simulink model "NHTSA_LDW_Curved_dashed_right_cs"  (Simulink 7.6)
settings: Solver=ode5  SolverMode=SingleTasking  StartTime=0.0  StopTime=10  FixedStep=1/100  RelTol=1e-3
model workspace (MAT data in the model file):
  mbox_table : struct (value not decoded)
  model_closed = 0
  sim_status = 0
PreLoadFcn:
  | check_NUTS_defined;
  | 
  | assignin('base',['model_closed_' bdroot],false);
  | 
  | if exist('LDW_mask_sfun.mexw64')==3
  | delete LDW_mask_sfun.mexw64;
  | end
  | 
  | if exist('LDW_mask_sfun.mexw32') ==3
  | delete LDW_mask_sfun.mexw32;
  | end
  | 
  | switch version('-release')
  | case {'2010a', '2010b', '2011a'}
  | addpath('../includes_LKAS/includes_LKAS_2010a');
  | case {'2011b', '2012a', '2012b'}
  | addpath('../includes_LKAS/includes_LKAS_2011b');
  | otherwise
  | addpath('../includes_LKAS/includes_LKAS_2011b');
  | end
InitFcn:
  | PreScanExperimentInitFcn(bdroot)
StopFcn:
  | PreScanExperimentStopFcn(bdroot)
undefined symbols (not defined in the file): DiscIntNeverNeededParam, InitImageOutputDir, x_ini_VRML, y_ini_VRML, z_ini_VRML
libraries: simulink x22, PreScanSimulinkLibrary x7, simulink_extras x6, dspsnks4 x2, PreScanUsefulBlocks x2, simulink_need_slupdate x1
(part 1 of 5)
CloseFcn:
  | evalin('base',['clear model_closed_' bdroot]);
  | 
  | set(0, 'ShowHiddenHandles', 'on')
  | 
  | try
  |     close (PlotSpeed)
  | end
  | 
  | try
  |     close(findobj('Name','Filtered'))
  | end
  | 
  | try
  |     close(findobj('Name','Results'))
  | end
  | 
  | set(0, 'ShowHiddenHandles', 'off')
settings Model: Creator=PRESCAN  LastModifiedBy=buildbot
settings OptimizationCC: InitFltsAndDblsToZero=on
settings DebuggingCC: SaveWithParameterizedLinksMsg=none  SignalResolutionControl=TryResolveAllWithWarning  SolverPrmCheckMsg=none  MultiTaskDSMMsg=warning  MultiTaskCondExecSysMsg=none
settings SFSimCC: SimParseCustomCode=off
settings RTWCC: IncludeERTFirstTime=on
settings GRTTargetCC: TargetFcnLib=ansi_tfl_tmw.mat

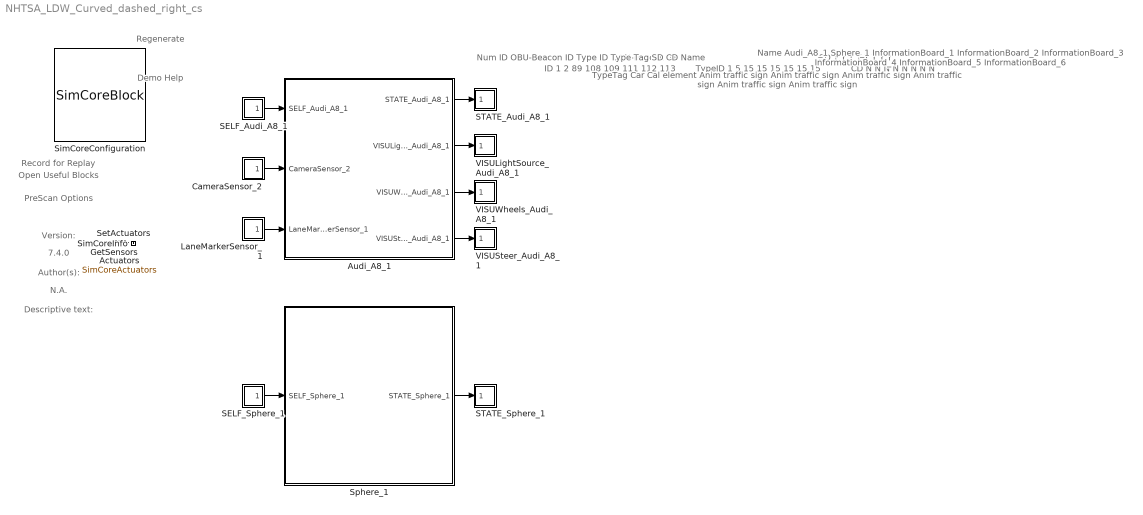
== system NHTSA_LDW_Curved_dashed_right_cs ==
  note: Demo Help
  note: Regenerate
  note: Record for Replay
  note: Open Useful Blocks
  note: PreScan Options
  note: Version:
  note: 7.4.0
  note: Author(s):
  note: N.A.
  note: Descriptive text:
  note: ID
      |
      | 1
      | 2
      | 89
      | 108
      | 109
      | 111
      | 112
      | 113
  note: OBU-Beacon ID
  note: TypeID
      |
      | 1
      | 5
      | 15
      | 15
      | 15
      | 15
      | 15
      | 15
  note: TypeTag
      |
      | Car
      | Cal element
      | Anim traffic sign
      | Anim traffic sign
      | Anim traffic sign
      | Anim traffic sign
      | Anim traffic sign
      | Anim traffic sign
  note: SD
      |
      | Y
      | Y
      | Y
      | Y
      | Y
      | Y
      | Y
      | Y
  note: CD
      |
      | N
      | N
      | N
      | N
      | N
      | N
      | N
      | N
  note: Name
      |
      | Audi_A8_1
      | Sphere_1
      | InformationBoard_1
      | InformationBoard_2
      | InformationBoard_3
      | InformationBoard_4
      | InformationBoard_5
      | InformationBoard_6
  note: Num ID OBU-Beacon ID Type ID Type Tag SD CD Name
  Actuators : DataStoreMemory  Tag=Actuators  DataStoreName=SimCoreActuators  InitialValue=zeros(258,1)
      settings: DeleteFcn=PreScanBlockDeleteFcn;
  Audi_A8_1 : Subsystem  Tag=WorldObjectSubSystem  InitFcn=UniqueId = '253';
      mask Display: image(imread('Audi_A8.jpg'));color('white');text(0,0,' ID=1\n')
  CameraSensor_2 : Subsystem  Tag=CameraSensor  Priority=3
      settings: DeleteFcn=PreScanBlockDeleteFcn;
      mask Type: PreScan Source Block: Camera Sensor
      mask Description: The Camera Sensor provides a color or monochrome image.
      mask Help: eval('openHelp(457)')
      mask Display: image(imread('CameraSensor.png'))
  GetSensors : Subsystem  Tag=GetSensors  Priority=2  mask(PreScan Simulation Core Block){NrOfSensors=16, TimeStep=1/100}
      mask prompts: NrOfSensors "Number of sensor values"; TimeStep "Timestep [s]"
      mask help:
      | Please do not remove this block from the PreScan compilation sheet,
      | as it contains essential configuration parameters for a PreScan simulation.
      settings: DeleteFcn=PreScanBlockDeleteFcn;
  LaneMarkerSensor_1 : Subsystem  Tag=LaneMarkerSensor  Priority=3
      settings: DeleteFcn=PreScanBlockDeleteFcn;
      mask Type: PreScan Source Block: Lane Marker Sensor
      mask Description: The Lane Marker Sensor provides information relating the sensor to the lane markers on the road.
      mask Help: eval('openHelp(457)')
      mask Display: image(imread('LaneMarkerSensorSL.png'))
  SELF_Audi_A8_1 : Subsystem  Tag=SELF  Priority=3  mask(PreScan Source Block: SELF){PortName=SELF_Audi_A8_1, PortIndex=0, PortWidth=8, TimeStep=1/100}
      mask prompts: PortName "Auto-Assigned: Port Name [-]"; PortIndex "Auto-Assigned: Port Index [-]"; PortWidth "Auto-Assigned: Port Dimensions"; TimeStep "Auto-Assigned: Upload Period [s]"
      mask help:
      | The SELF port shows (state) information of the actor itself. The outputs are position in the experiment's axis system and the GPS coordinates, and the object's absolute velocity and compass heading.
      |
      | For more information, please click Help.
      settings: DeleteFcn=PreScanBlockDeleteFcn;
      mask Help: eval('openHelp(462)')
      mask Display: image(imread('GPS.png'))
  SELF_Sphere_1 : Subsystem  Tag=SELF  Priority=3  mask(PreScan Source Block: SELF){PortName=SELF_Sphere_1, PortIndex=8, PortWidth=8, TimeStep=1/100}
      mask prompts: PortName "Auto-Assigned: Port Name [-]"; PortIndex "Auto-Assigned: Port Index [-]"; PortWidth "Auto-Assigned: Port Dimensions"; TimeStep "Auto-Assigned: Upload Period [s]"
      mask help:
      | The SELF port shows (state) information of the actor itself. The outputs are position in the experiment's axis system and the GPS coordinates, and the object's absolute velocity and compass heading.
      |
      | For more information, please click Help.
      settings: DeleteFcn=PreScanBlockDeleteFcn;
      mask Help: eval('openHelp(462)')
      mask Display: image(imread('GPS.png'))
  STATE_Audi_A8_1 : Subsystem  Tag=State  Priority=0  mask(PreScan Sink Block: State){x0=25.564167022705078, y0=61.75, z0=0.55, Roll0=0, Pitch0=0, Yaw0=0, TimeStep=1/100}
      mask prompts: x0 "Ini x-position VEHICLE wrt GLOBAL axis system [m]"; y0 "Ini y-position VEHICLE wrt GLOBAL axis system [m]"; z0 "Ini z-position VEHICLE wrt GLOBAL axis system [m]"; Roll0 "Ini roll-angle BODY wrt VEHICLE axis system [deg]"; Pitch0 "Ini pitch-angle BODY wrt VEHICLE axis system [deg]"; Yaw0 "Ini yaw-angle VEHICLE wrt GLOBAL axis system [deg]"; TimeStep "Time Step [s]"
      mask help:
      | The Actor State contains a vector signal of size (9x1), containing the following signals:
      |
      | -  Position                  (x,y,z)                                     [m]
      | -  Velocity                  (vx,vy,vz)                               [m/s]
      | -  Angles                    (Roll, Pitch, Yaw)                   [rad]
      |
      | The Actor state is defined in the global axis system.
      | The state is superponed on the Initial position defined in the GUI.
      |
      | For more information, please click Help.
      settings: DeleteFcn=PreScanBlockDeleteFcn;
      mask Help: eval('openHelp(222)')
      mask Display: image(imread('State.png'))
  STATE_Sphere_1 : Subsystem  Tag=State  Priority=0  mask(PreScan Sink Block: State){x0=25.564167022705078, y0=61.75, z0=0, Roll0=0, Pitch0=0, Yaw0=0, TimeStep=1/100}
      mask prompts: x0 "Ini x-position VEHICLE wrt GLOBAL axis system [m]"; y0 "Ini y-position VEHICLE wrt GLOBAL axis system [m]"; z0 "Ini z-position VEHICLE wrt GLOBAL axis system [m]"; Roll0 "Ini roll-angle BODY wrt VEHICLE axis system [deg]"; Pitch0 "Ini pitch-angle BODY wrt VEHICLE axis system [deg]"; Yaw0 "Ini yaw-angle VEHICLE wrt GLOBAL axis system [deg]"; TimeStep "Time Step [s]"
      mask help:
      | The Actor State contains a vector signal of size (9x1), containing the following signals:
      |
      | -  Position                  (x,y,z)                                     [m]
      | -  Velocity                  (vx,vy,vz)                               [m/s]
      | -  Angles                    (Roll, Pitch, Yaw)                   [rad]
      |
      | The Actor state is defined in the global axis system.
      | The state is superponed on the Initial position defined in the GUI.
      |
      | For more information, please click Help.
      settings: DeleteFcn=PreScanBlockDeleteFcn;
      mask Help: eval('openHelp(222)')
      mask Display: image(imread('State.png'))
  SetActuators : Subsystem  Tag=SetActuators  Priority=1  mask(PreScan Simulation Core Block){TimeStep=1/100, NrOfActuators=258}
      mask prompts: TimeStep "Timestep [s]"; NrOfActuators "Number of actuator values"
      mask help:
      | Please do not remove this block from the PreScan compilation sheet,
      | as it contains essential configuration parameters for a PreScan simulation.
      settings: DeleteFcn=PreScanBlockDeleteFcn;
  SimCoreConfiguration : M-S-Function  Tag=SimCoreConfiguration  Description=7FB4F5B2D4E922D3E47F677EE9558725FCFBD13CCF8702ED0EADB85902E5BDE3  FunctionName=SimCoreBlock  Parameters=ExperimentXML PortsXML SimulationCore HostName CheckStart EnableLog RfR EnableGPUAccel ShowComputationTime  mask(PreScan Simulation Core Configurator){SimulationCore=NUTS, HostName=0, CheckStart=0, prescanversion='7.4.0', EnableLog=off, RfR=0, EnableGPUAccel=off, ShowComputationTime=off}
      mask prompts: SimulationCore "Simulation Core"; HostName "Simulation Host"; CheckStart "Show START Dialog"; prescanversion "PreScan Version"; EnableLog "Create TA Log"; RfR "Record for Replay"; EnableGPUAccel "Enable GPU Acceleration"; ShowComputationTime "Show ComputationTime Scope"
      mask help:
      | Please do not remove this block from the PreScan compilation sheet,
      | as it contains essential configuration parameter for a PreScan simulation.
      mask init:
      | model = bdroot;
      | ExperimentXML = [model(1:end-3) '.pex'];
      | PortsXML = [model '_ports.pcd'];
      settings: DeleteFcn=PreScanBlockDeleteFcn;  ModelCloseFcn=assignin('base',['model_closed_' bdroot],true);
      mask Help: eval('openHelp(812)')
      mask Display: image(imread('prescanlogo.ico'))
  SimCoreInfo : Subsystem  Tag=SimCoreInfo
  Sphere_1 : Subsystem  Tag=WorldObjectSubSystem  InitFcn=UniqueId = '274';
      mask Display: image(imread('Sphere.jpg'));color('white');text(0,0,' ID=2\n')
  VISULightSource_Audi_A8_1 : Subsystem  Tag=VisuLightSource  Priority=0
      settings: DeleteFcn=PreScanBlockDeleteFcn;
      mask Type: PreScan Sink Block: VisuLightSource
      mask Description:
      | The VisuLightSource block provides a way to animate Light Sources of the indicator, braking, fog and main lights of a vehicle.
      | 
      | For more information, please click Help.
      mask Help: eval('openHelp(223)')
      mask Display: image(imread('RearLight.png'))
  VISUSteer_Audi_A8_1 : Subsystem  Tag=VisuSteer  Priority=0
      settings: DeleteFcn=PreScanBlockDeleteFcn;
      mask Type: PreScan Sink Block: VisuSteer
      mask Description:
      | The VisuSteer block provides a way to adapt the orientation of the steering column and steering wheel of a vehicle.
      | 
      | For more information, please click Help.
      mask Help: eval('openHelp(223)')
      mask Display: image(imread('steeringwheel.png'))
  VISUWheels_Audi_A8_1 : Subsystem  Tag=VisuWheels  Priority=0
      settings: DeleteFcn=PreScanBlockDeleteFcn;
      mask Type: PreScan Sink Block: VisuWheels
      mask Description:
      | The VisuWheels block provides a way to animate the wheels of a vehicle, with steering, rotation (because of velocity) and z-displacement.
      | 
      | For more information, please click Help.
      mask Help: eval('openHelp(223)')
      mask Display: image(imread('wheel.png'))
  wires:
  Audi_A8_1/1(STATE_Audi_A8_1) -> STATE_Audi_A8_1/1(State)
  SELF_Audi_A8_1/1(U) -> Audi_A8_1/1(SELF_Audi_A8_1)
  CameraSensor_2/1(U1) -> Audi_A8_1/2(CameraSensor_2)
  LaneMarkerSensor_1/1(U) -> Audi_A8_1/3(LaneMarkerSensor_1)
  Audi_A8_1/2(VISULightSource_Audi_A8_1) -> VISULightSource_Audi_A8_1/1(Lights)
  Audi_A8_1/3(VISUWheels_Audi_A8_1) -> VISUWheels_Audi_A8_1/1(Wheels)
  Audi_A8_1/4(VISUSteer_Audi_A8_1) -> VISUSteer_Audi_A8_1/1(Steer)
  Sphere_1/1(STATE_Sphere_1) -> STATE_Sphere_1/1(State)
  SELF_Sphere_1/1(U) -> Sphere_1/1(SELF_Sphere_1)
  SetActuators/1(dummy) -> GetSensors/1(dummy)

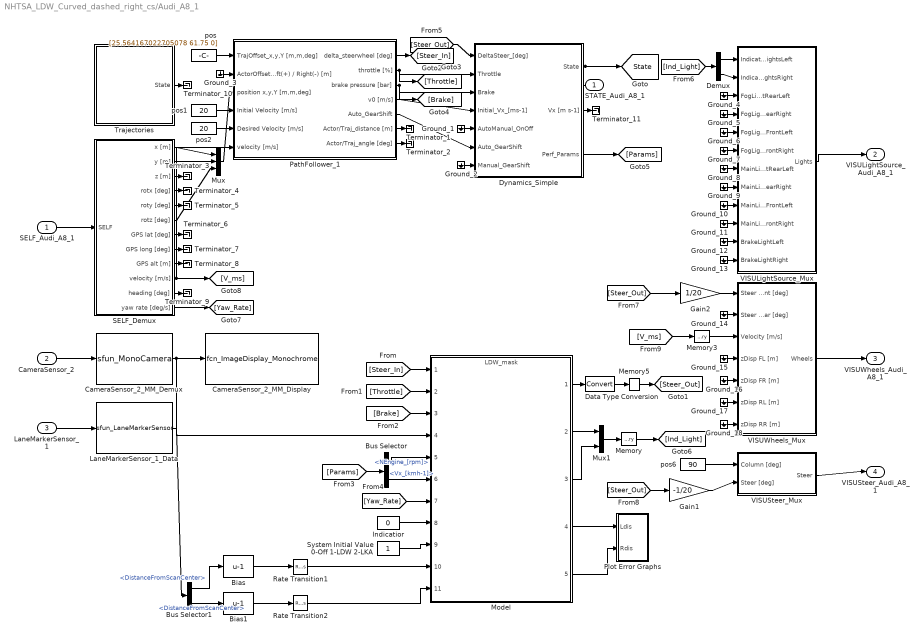
== system NHTSA_LDW_Curved_dashed_right_cs/Audi_A8_1 ==
  SELF_Audi_A8_1 : Inport  Tag=SELFInport
  CameraSensor_2 : Inport  Tag=CameraSensorInport  Port=2  SampleTime=1/50
  LaneMarkerSensor_1 : Inport  Tag=LaneMarkerSensorInport  Port=3  SampleTime=1/10
  Bias : Bias  Bias=-1
  Bias1 : Bias  Bias=-1
  Bus Selector : BusSelector  OutputSignals=NEngine_[rpm],Vx_[kmh-1]
  Bus Selector1 : BusSelector  OutputSignals=ScanAtDistance1.LeftLaneIntersection1.DistanceFromScanCenter,ScanAtDistance1.RightLaneIntersection1.DistanceFromScanCenter
  CameraSensor_2_MM_Demux : S-Function  Tag=CameraSensor_Monochrome_Demux  FunctionName=sfun_MonoCamera  Parameters=[VerticalResolution HorizontalResolution] FrameRate SensorName CameraType SharedMemTag SharedMemRightTag DataType HasInputPort  EnableBusSupport=off  mask{HorizontalResolution=500, VerticalResolution=375, FrameRate=50, SensorName=CameraSensor_2, CameraType=Mono, SharedMemTag=CameraSensor_2_monoBeam_viewer_RGB, SharedMemRightTag=CameraSensor_2_StereoRight_viewer_RGB, DataType=uint8, HasInputPort=1}
      mask prompts: HorizontalResolution "User Specified: Horizontal Resolution [pixels]"; VerticalResolution "User Specified: Vertical Resolution [pixels]"; FrameRate "User Specified: Frame Rate [Hz]"; SensorName "User Specified: Camera Sensor Name"; CameraType "Camera type"; SharedMemTag "Tag for shared memory for main img"; SharedMemRightTag "Tag for shared memory for right img"; DataType "Image data type"; HasInputPort "Has input port"
      mask init:
      | if CameraType==1
      |     CameraTypeName='MONO';
      |     CameraPort1Name='I';
      |     CameraPort2Name='I';
      |     PortNumber=0;
      | else
      |     CameraTypeName='STEREO';
      |     CameraPort1Name='Left';
      |     CameraPort2Name='Right';
      |     PortNumber=1;
      | end
      settings: DeleteFcn=PreScanBlockDeleteFcn;
      mask StyleString: edit,edit,edit,edit,popup(Mono|Stereo),edit,edit,popup(uint8|single),edit
      mask Display:
      | fprintf('%s CAMERA:\n Monochrome\n%s \n V: %d x %d \n %d fps',CameraTypeName,SensorName,VerticalResolution,HorizontalResolution,FrameRate)
      | port_label('output',1,CameraPort1Name)
      | port_label('output',PortNumber+1,CameraPort2Name)
  CameraSensor_2_MM_Display : M-S-Function  Tag=CameraSensor_Monochrome_Display  InitFcn=InitImageOutputDir(gcb);  FunctionName=fcn_ImageDisplay_Monochrome  Parameters=SensorName EnableDisplay EnablePosition DisplayPosition FigureHandle SaveResults BitmapFormat TempOutputDir CameraType DataType  mask(PreScan Monochrome Display Block){SensorName=CameraSensor_2, EnableDisplay=on, EnablePosition=off, DisplayPosition=[10 10 500 375], FigureHandle=100, SaveResults=off, Format=PNG, TempOutputDir=0, CameraType=Mono, DataType=uint8}
      mask prompts: SensorName "User Specified: Title of Display"; EnableDisplay "Active"; EnablePosition "Set Display window position"; DisplayPosition "Display window position [xpos ypos width height]"; FigureHandle "Unique handle"; SaveResults "Save results"; TempOutputDir "OutputDir"; CameraType "Camera Type"; DataType "Image Data Type"
      mask help: This block displays the Monochrome output of a PreScan camera sensor.
      mask init:
      | if EnableDisplay
      |     EnableString='';
      |     EnableColor='gray';
      | else
      |     EnableString='INACTIVE';
      |     EnableColor='red';
      | end
      | switch Format
      |     case 1
      |         BitmapFormat = 'png';
      |     case 2
      |         BitmapFormat = 'bmp';
      |     case 3
      |         BitmapFormat = 'jpg';
      | end
      | if CameraType==1
      |     CameraTypeName='MONO';
      |     PortNumber=0;
      | else
      |     CameraTypeName='STEREO';
      |     PortNumber=1;
      | end
      settings: CopyFcn=CopyFcnDisplay  DeleteFcn=PreScanBlockDeleteFcn;  ModelCloseFcn=fcn_ImageDisplay_ModelCloseFcn
      mask Help: eval('openHelp(457)')
      mask StyleString: edit,checkbox,checkbox,edit,edit,checkbox,popup(PNG|BMP|JPG),edit,popup(Mono|Stereo),popup(uint8|single)
      mask CallbackString:
      | ||MV=get_param(gcb,'MaskVisibilities');
      | if strcmp(get_param(gcb,'EnablePosition'),'on')
      |     MV{4}='on';
      | else
      |     MV{4}='off';
      | end
      | set_param(gcb,'MaskVisibilities',MV);|||||||
      mask Display:
      | color(EnableColor);
      | fprintf('%s\n DISPLAY:\n Monochrome\n %s',EnableString,SensorName)
      | port_label('input',1,'I')
      | port_label('input',PortNumber+1,'I')
  Data Type Conversion : DataTypeConversion
  Demux : Demux  Outputs=2
  Dynamics_Simple : Subsystem  Tag=Simple_Vehicle_Dynamics  mask(PreScan Block: Simple Dynamics){Migrate=off, TimeStep=1/100, ComputationMode=Continuous_Time}
      mask prompts: Migrate "Migrate. During migration this block will be replaced by a newer one."; TimeStep "Auto assigned: Time Step [s]"; ComputationMode "Computation mode:"
      mask help:
      | The Simple Dynamics Model is selected in the GUI to simulate vehicle dynamics behavior.
      |
      | The Simple Dynamics Model is completely open to the user. The parameters of this model can be set in the Simple Dynamics dialog in the GUI.
      |
      | For more information, please click Help.
      mask init:
      | p = SimpleDyn_pars;
      settings: DeleteFcn=PreScanBlockDeleteFcn;
      mask Help: eval('openHelp(220)')
      mask Display:
      | image(imread('SimpleDyn.png'))
      | port_label('input', 1, '{\delta}_S_t_ _e_e_r [deg]','texmode','on')
      | port_label('input', 2, 'Throttle [%]')
      | port_label('input', 3, 'Brake Pres [bar]')
      | port_label('input', 4, 'V_0 [ms-1]','texmode','on')
      | port_label('input', 5, 'Auto=[0]/Manual=[1]')
      | port_label('input', 6, 'Auto_GearShift')
      | port_label('input', 7, 'Manual_GearShift')
      | port_label('output', 1, 'State')
      | port_label('output', 2, 'Vx [ms-1]')
      | port_label('output', 3, 'Perf Params')
  Gain1 : Gain  Gain=-1/20
  Gain2 : Gain  Gain=1/20
  Ground_{1..18} (18 alike) : Ground
  Indicatior : Constant  Value=0  OutDataTypeStr=uint8
  LaneMarkerSensor_1_Data : S-Function  Tag=LaneMarkerSensor_Data  LoadFcn=load('LaneMarkerSensorBusses.mat');  FunctionName=sfun_LaneMarkerSensor  Parameters=[VerticalResolution HorizontalResolution] FrameRate SensorName OutputReferenceImage SharedMemTag SharedMemDataTag  EnableBusSupport=on  mask{HorizontalResolution=320, VerticalResolution=240, FrameRate=10, SensorName=LaneMarkerSensor_1, OutputReferenceImage=off, SharedMemTag=LaneMarkerSensor_1_monoBeam_viewer_RGB, SharedMemDataTag=LaneMarkerSensor_1_monoBeam_viewer_LMS_Data}
      mask prompts: HorizontalResolution "User Specified: Horizontal Resolution [pixels]"; VerticalResolution "User Specified: Vertical Resolution [pixels]"; FrameRate "User Specified: Frame Rate [Hz]"; SensorName "User Specified: Lane Marker Sensor Name"; OutputReferenceImage "User Specified: Output Reference Image"; SharedMemTag "Tag for shared memory for lane marker img"; SharedMemDataTag "Tag for shared memory data"
      mask init:
      | DataPort = 1;
      | if OutputReferenceImage==1
      |     Rport = 2;
      |     Gport = 3;
      |     Bport = 4;
      |     RportName = 'Ref. Image R';
      |     GportName = 'Ref. Image G';
      |     BportName = 'Ref. Image B';
      | else
      |     Rport = 1;
      |     Gport = 1;
      |     Bport = 1;
      |     RportName = '';
      |     GportName = '';
      |     BportName = '';
      | end
      settings: DeleteFcn=PreScanBlockDeleteFcn;
      mask Display:
      | port_label('output',DataPort,'Detection Data')
      | port_label('output',Rport,RportName)
      | port_label('output',Gport,GportName)
      | port_label('output',Bport,BportName)
  Memory : Memory
  Memory3 : Memory
  Memory5 : Memory
  Model : ModelReference  ModelNameDialog=LDW_mask  SimulationMode=Normal  ModelReferenceVersion=1.416  CopyOfModelName=LDW_mask
  Mux : Mux  Inputs=3
  Mux1 : Mux  Inputs=2
  PathFollower_1 : Subsystem  Tag=pathFollower  mask(PreScan Block: Path Follower){Migrate=on, FileName='Trajectory_1.mat', TunableSteeringGain=1, XShifting_wrt_COG=0}
      mask prompts: Migrate "Migrate. During migration this block will be replaced by a newer one."; FileName "Trajectory Name"; TunableSteeringGain "TunableSteeringGain [-]"; XShifting_wrt_COG "XShifting_wrt_COG [m]"
      mask help:
      | The Path Follower Model is selected in the GUI to simulate driver behavior.
      |
      | For more information, please click Help.
      mask init:
      | load(['trajectories/',eval(FileName)])
      | traject=trajectory';
      | 
      | Traj_x=traject(:,2);
      | Traj_y=traject(:,3);
      | Traj_z=traject(:,4);
      | Traj_vx=traject(:,8);
      | Traj_vy=traject(:,9);
      | Traj_vz=traject(:,10);
      mask Help: eval('openHelp(232)')
  Plot Error Graphs : Subsystem
  Rate Transition1 : RateTransition
  Rate Transition2 : RateTransition
  SELF_Demux : Subsystem  Tag=DemuxSELF
      settings: DeleteFcn=PreScanBlockDeleteFcn;
      mask Type: PreScan Demux Block:
      mask Display:
      | port_label('output',1,'x [m]')
      | port_label('output',2,'y [m]')
      | port_label('output',3,'z [m]','texmode','on')
      | port_label('output',4,'Rotx [deg]','texmode','on')
      | port_label('output',5,'Roty [deg]','texmode','on')
      | port_label('output',6,'Rotz [deg]','texmode','on')
      | port_label('output',7,'GPS lat [deg]','texmode','on')
      | port_label('output',8,'GPS long [deg]','texmode','on')
      | port_label('output',9,'GPS alt [m]','texmode','on')
      | port_label('output',10,'Velocity [m/s]')
      | port_label('output',11,'Heading [deg]')
      | port_label('output',12,'Yaw rate [deg/s]')
  System Initial Value 0-Off 1-LDW 2-LKA : Constant
  Terminator_{1..11} (11 alike) : Terminator
  Trajectories : Subsystem  Tag=Trajectories
      settings: DeleteFcn=PreScanBlockDeleteFcn;
      mask Type: PreScan Source Block: Trajectories
      mask Description:
      | The Trajectory block contains the trajectories defined in the PreScan Experiment Editor. The output of the trajectory block is the (vehicle) State.
      | 
      | For more information, please click Help.
      mask Help: eval('openHelp(312)')
      mask Display: image(imread('Trajectory.png'));
  VISULightSource_Mux : Subsystem  Tag=MuxLightSource
      settings: DeleteFcn=PreScanBlockDeleteFcn;
      mask Type: PreScan Mux Block:
  VISUSteer_Mux : Subsystem  Tag=MuxSteer
      settings: DeleteFcn=PreScanBlockDeleteFcn;
      mask Type: PreScan Mux Block:
  VISUWheels_Mux : Subsystem  Tag=MuxWheels  mask(PreScan Mux Block:){TimeStep=1/100}
      mask prompts: TimeStep "Auto Assigned: Time Step [s]"
      settings: DeleteFcn=PreScanBlockDeleteFcn;
  pos : Constant  Tag=pos  Value=[25.564167022705078 61.75 0]
  pos1 : Constant  Tag=pos  Value=20
  pos2 : Constant  Tag=pos  Value=20
  pos6 : Constant  Tag=pos  Value=90
  STATE_Audi_A8_1 : Outport  Tag=StateOutport
  VISULightSource_Audi_A8_1 : Outport  Tag=VisuLightsOutport  Port=2  SampleTime=1/100
  VISUWheels_Audi_A8_1 : Outport  Tag=VisuWheelsOutport  Port=3  SampleTime=1/100
  VISUSteer_Audi_A8_1 : Outport  Tag=VisuSteerOutport  Port=4  SampleTime=1/100
  tag scope: State=global
  wires:
  Bus Selector1/1 -> Bias/1  "<DistanceFromScanCenter>"
  Bus Selector1/2 -> Bias1/1  "<DistanceFromScanCenter>"
  Bias/1 -> Rate Transition1/1
  Bias1/1 -> Rate Transition2/1
  Model/1 -> Data Type Conversion/1
  Model/4 -> Plot Error Graphs/1(Ldis)
  Model/5 -> Plot Error Graphs/2(Rdis)
  Indicatior/1 -> Model/8
  System Initial Value 0-Off 1-LDW 2-LKA/1 -> Model/9
  Bus Selector/1 -> Model/5  "<NEngine_[rpm]>"
  Bus Selector/2 -> Model/6  "<Vx_[kmh-1]>"
  Rate Transition1/1 -> Model/10
  Rate Transition2/1 -> Model/11
  Data Type Conversion/1 -> Memory5/1
  Model/2 -> Mux1/1
  Model/3 -> Mux1/2
  Mux1/1 -> Memory/1
  Memory/1 -> [Ind_Light]
  [Steer_In] -> Model/1
  [Throttle] -> Model/2
  [Brake] -> Model/3
  [Params] -> Bus Selector/1
  [Yaw_Rate] -> Model/7
  [Steer_Out] -> Gain1/1
  [V_ms] -> Memory3/1
  Memory5/1 -> [Steer_Out]
  [Steer_Out] -> Gain2/1
  [Ind_Light] -> Demux/1
  pos/1 -> PathFollower_1/1(TrajOffset_x,y,Y [m,m,deg])
  SELF_Audi_A8_1/1 -> SELF_Demux/1(SELF)
  CameraSensor_2_MM_Demux/1 -> CameraSensor_2_MM_Display/1, Model/4
  CameraSensor_2/1 -> CameraSensor_2_MM_Demux/1
  LaneMarkerSensor_1/1 -> LaneMarkerSensor_1_Data/1
  VISULightSource_Mux/1(Lights) -> VISULightSource_Audi_A8_1/1
  VISUWheels_Mux/1(Wheels) -> VISUWheels_Audi_A8_1/1
  VISUSteer_Mux/1(Steer) -> VISUSteer_Audi_A8_1/1
  PathFollower_1/4(v0 [m/s]) -> Dynamics_Simple/4(Initial_Vx_[ms-1])
  PathFollower_1/5(Auto_GearShift) -> Dynamics_Simple/6(Auto_GearShift)
  PathFollower_1/2(throttle [%]) -> Dynamics_Simple/2(Throttle), [Throttle]
  PathFollower_1/3(brake pressure [bar]) -> Dynamics_Simple/3(Brake), [Brake]
  Dynamics_Simple/1(State) -> STATE_Audi_A8_1/1, [State]
  SELF_Demux/1(x [m]) -> Mux/1
  SELF_Demux/2(y [m]) -> Mux/2
  SELF_Demux/6(rotz [deg]) -> Mux/3
  Mux/1 -> PathFollower_1/3(position x,y,Y [m,m,deg])
  pos1/1 -> PathFollower_1/4(Initial Velocity [m/s])
  pos2/1 -> PathFollower_1/5(Desired Velocity [m/s])
  SELF_Demux/10(velocity [m/s]) -> PathFollower_1/6(velocity [m/s]), [V_ms]
  LaneMarkerSensor_1_Data/1 -> Bus Selector1/1
  Memory3/1 -> VISUWheels_Mux/3(Velocity [m/s])
  Gain2/1 -> VISUWheels_Mux/1(Steer Angle Front [deg])
  pos6/1 -> VISUSteer_Mux/1(Column [deg])
  Gain1/1 -> VISUSteer_Mux/2(Steer [deg])
  Demux/1 -> VISULightSource_Mux/1(IndicatorLightsLeft)
  Demux/2 -> VISULightSource_Mux/2(IndicatorLightsRight)
  [Steer_Out] -> Dynamics_Simple/1(DeltaSteer_[deg])
  SELF_Demux/12(yaw rate [deg/s]) -> [Yaw_Rate]
  Dynamics_Simple/3(Perf_Params) -> [Params]
  PathFollower_1/1(delta_steerwheel [deg]) -> [Steer_In]
  Dynamics_Simple/2(Vx [m s-1]) -> Terminator_11/1
  Ground_1/1 -> Dynamics_Simple/5(AutoManual_OnOff)
  Ground_2/1 -> Dynamics_Simple/7(Manual_GearShift)
  Ground_3/1 -> PathFollower_1/2(ActorOffset_Left(+) / Right(-) [m])
  PathFollower_1/6(Actor/Traj_distance [m]) -> Terminator_1/1
  PathFollower_1/7(Actor/Traj_angle [deg]) -> Terminator_2/1
  SELF_Demux/3(z [m]) -> Terminator_3/1
  SELF_Demux/4(rotx [deg]) -> Terminator_4/1
  SELF_Demux/5(roty [deg]) -> Terminator_5/1
  SELF_Demux/7(GPS lat [deg]) -> Terminator_6/1
  SELF_Demux/8(GPS long [deg]) -> Terminator_7/1
  SELF_Demux/9(GPS alt [m]) -> Terminator_8/1
  SELF_Demux/11(heading [deg]) -> Terminator_9/1
  Trajectories/1(State) -> Terminator_10/1
  Ground_4/1 -> VISULightSource_Mux/3(FogLightRearLeft)
  Ground_5/1 -> VISULightSource_Mux/4(FogLightRearRight)
  Ground_6/1 -> VISULightSource_Mux/5(FogLightFrontLeft)
  Ground_7/1 -> VISULightSource_Mux/6(FogLightFrontRight)
  Ground_8/1 -> VISULightSource_Mux/7(MainLightRearLeft)
  Ground_9/1 -> VISULightSource_Mux/8(MainLightRearRight)
  Ground_10/1 -> VISULightSource_Mux/9(MainLightFrontLeft)
  Ground_11/1 -> VISULightSource_Mux/10(MainLightFrontRight)
  Ground_12/1 -> VISULightSource_Mux/11(BrakeLightLeft)
  Ground_13/1 -> VISULightSource_Mux/12(BrakeLightRight)
  Ground_14/1 -> VISUWheels_Mux/2(Steer Angle Rear [deg])
  Ground_15/1 -> VISUWheels_Mux/4(zDisp FL [m])
  Ground_16/1 -> VISUWheels_Mux/5(zDisp FR [m])
  Ground_17/1 -> VISUWheels_Mux/6(zDisp RL [m])
  Ground_18/1 -> VISUWheels_Mux/7(zDisp RR [m])

== system NHTSA_LDW_Curved_dashed_right_cs/CameraSensor_2 ==
  Demux : Demux  Outputs=[1 -1]
  Terminator : Terminator
  U1 : Outport
  wires:
  Demux/2 -> Terminator/1
  Demux/1 -> U1/1
  [SimCoreSensors] -> Demux/1

== system NHTSA_LDW_Curved_dashed_right_cs/GetSensors ==
  dummy : Inport
  GetSensors : M-S-Function  FunctionName=GetSensorsBlock  Parameters=TimeStep NrOfSensors
  tag scope: SimCoreSensors=global
  wires:
  GetSensors/1 -> [SimCoreSensors]
  dummy/1 -> GetSensors/1

== system NHTSA_LDW_Curved_dashed_right_cs/LaneMarkerSensor_1 ==
  Demux : Demux  Outputs=[1 -1]
  Terminator : Terminator
  U : Outport
  wires:
  Demux/2 -> Terminator/1
  Demux/1 -> U/1
  [SimCoreSensors] -> Demux/1

== system NHTSA_LDW_Curved_dashed_right_cs/SELF_Audi_A8_1 ==
  Selector : Selector  IndexMode=Zero-based  IndexOptions=Starting index (dialog)  Indices=PortIndex  OutputSizes=PortWidth(1)
  U : Outport
  wires:
  Selector/1 -> U/1
  [SimCoreSensors] -> Selector/1

== system NHTSA_LDW_Curved_dashed_right_cs/SELF_Sphere_1 ==
  Selector : Selector  IndexMode=Zero-based  IndexOptions=Starting index (dialog)  Indices=PortIndex  OutputSizes=PortWidth(1)
  U : Outport
  wires:
  Selector/1 -> U/1
  [SimCoreSensors] -> Selector/1

== system NHTSA_LDW_Curved_dashed_right_cs/STATE_Audi_A8_1 ==
  State : Inport  SampleTime=TimeStep
  Acceleration : Subsystem  mask(ToSensorWorld){PortName=Acceleration_Audi_A8_1, PortIndex=6, PortWidth=3, TimeStep=1/100}
      mask prompts: PortName "Port Name [-]"; PortIndex "Index [-]"; PortWidth "Port Dimensions [-]"; TimeStep "Upload Period [s]"
      mask help: Sends signal(s) from Simulink to the Sensor World
      mask Help:
      | Sends signal(s) from Simulink to the Sensor World.
      | 
      | - Port Name [-]: specifies the name of the output terminal of the Simulink block.
      | - Index [-]: specifies the start position in the output vector sent to the Sensor World
      | - Port dimensions [-]: specifies the width (number of scalars) of the output port
      | - Upload period [s]: specifies the upload period (in seconds) of the port.
      mask Display: port_label('input', 1, PortName)
  Demux : Demux  Outputs=5
  Position : Subsystem  mask(ToSensorWorld){PortName=Position_Audi_A8_1, PortIndex=0, PortWidth=3, TimeStep=1/100}
      mask prompts: PortName "Port Name [-]"; PortIndex "Index [-]"; PortWidth "Port Dimensions [-]"; TimeStep "Upload Period [s]"
      mask help: Sends signal(s) from Simulink to the Sensor World
      mask Help:
      | Sends signal(s) from Simulink to the Sensor World.
      | 
      | - Port Name [-]: specifies the name of the output terminal of the Simulink block.
      | - Index [-]: specifies the start position in the output vector sent to the Sensor World
      | - Port dimensions [-]: specifies the width (number of scalars) of the output port
      | - Upload period [s]: specifies the upload period (in seconds) of the port.
      mask Display: port_label('input', 1, PortName)
  RPY : Subsystem  mask(ToSensorWorld){PortName=RPY_Audi_A8_1, PortIndex=9, PortWidth=3, TimeStep=1/100}
      mask prompts: PortName "Port Name [-]"; PortIndex "Index [-]"; PortWidth "Port Dimensions [-]"; TimeStep "Upload Period [s]"
      mask help: Sends signal(s) from Simulink to the Sensor World
      mask Help:
      | Sends signal(s) from Simulink to the Sensor World.
      | 
      | - Port Name [-]: specifies the name of the output terminal of the Simulink block.
      | - Index [-]: specifies the start position in the output vector sent to the Sensor World
      | - Port dimensions [-]: specifies the width (number of scalars) of the output port
      | - Upload period [s]: specifies the upload period (in seconds) of the port.
      mask Display: port_label('input', 1, PortName)
  Velocity : Subsystem  mask(ToSensorWorld){PortName=Velocity_Audi_A8_1, PortIndex=3, PortWidth=3, TimeStep=1/100}
      mask prompts: PortName "Port Name [-]"; PortIndex "Index [-]"; PortWidth "Port Dimensions [-]"; TimeStep "Upload Period [s]"
      mask help: Sends signal(s) from Simulink to the Sensor World
      mask Help:
      | Sends signal(s) from Simulink to the Sensor World.
      | 
      | - Port Name [-]: specifies the name of the output terminal of the Simulink block.
      | - Index [-]: specifies the start position in the output vector sent to the Sensor World
      | - Port dimensions [-]: specifies the width (number of scalars) of the output port
      | - Upload period [s]: specifies the upload period (in seconds) of the port.
      mask Display: port_label('input', 1, PortName)
  iniBODYAngles wrtVEH [rad] : Constant  Value=[Roll0 Pitch0 0]  SampleTime=TimeStep
  iniVEHAngles wrtGLOB [rad] : Constant  Value=[0 0 Yaw0]  SampleTime=TimeStep
  iniVEHposition wrtGLOB [m] : Constant  Value=[x0 y0 z0]  SampleTime=TimeStep
  state2FullState : PreScanSimulinkLibrary/state2FullState  SystemSampleTime=-1
  velRPY : Subsystem  mask(ToSensorWorld){PortName=velRPY_Audi_A8_1, PortIndex=12, PortWidth=3, TimeStep=1/100}
      mask prompts: PortName "Port Name [-]"; PortIndex "Index [-]"; PortWidth "Port Dimensions [-]"; TimeStep "Upload Period [s]"
      mask help: Sends signal(s) from Simulink to the Sensor World
      mask Help:
      | Sends signal(s) from Simulink to the Sensor World.
      | 
      | - Port Name [-]: specifies the name of the output terminal of the Simulink block.
      | - Index [-]: specifies the start position in the output vector sent to the Sensor World
      | - Port dimensions [-]: specifies the width (number of scalars) of the output port
      | - Upload period [s]: specifies the upload period (in seconds) of the port.
      mask Display: port_label('input', 1, PortName)
  wires:
  Demux/5 -> velRPY/1(Y)
  Demux/4 -> RPY/1(Y)
  Demux/3 -> Acceleration/1(Y)
  Demux/2 -> Velocity/1(Y)
  Demux/1 -> Position/1(Y)
  State/1 -> state2FullState/1
  state2FullState/1 -> Demux/1
  iniVEHposition wrtGLOB [m]/1 -> state2FullState/2
  iniBODYAngles wrtVEH [rad]/1 -> state2FullState/3
  iniVEHAngles wrtGLOB [rad]/1 -> state2FullState/4

== system NHTSA_LDW_Curved_dashed_right_cs/STATE_Sphere_1 ==
  State : Inport  SampleTime=TimeStep
  Acceleration : Subsystem  mask(ToSensorWorld){PortName=Acceleration_Sphere_1, PortIndex=249, PortWidth=3, TimeStep=1/100}
      mask prompts: PortName "Port Name [-]"; PortIndex "Index [-]"; PortWidth "Port Dimensions [-]"; TimeStep "Upload Period [s]"
      mask help: Sends signal(s) from Simulink to the Sensor World
      mask Help:
      | Sends signal(s) from Simulink to the Sensor World.
      | 
      | - Port Name [-]: specifies the name of the output terminal of the Simulink block.
      | - Index [-]: specifies the start position in the output vector sent to the Sensor World
      | - Port dimensions [-]: specifies the width (number of scalars) of the output port
      | - Upload period [s]: specifies the upload period (in seconds) of the port.
      mask Display: port_label('input', 1, PortName)
  Demux : Demux  Outputs=5
  Position : Subsystem  mask(ToSensorWorld){PortName=Position_Sphere_1, PortIndex=243, PortWidth=3, TimeStep=1/100}
      mask prompts: PortName "Port Name [-]"; PortIndex "Index [-]"; PortWidth "Port Dimensions [-]"; TimeStep "Upload Period [s]"
      mask help: Sends signal(s) from Simulink to the Sensor World
      mask Help:
      | Sends signal(s) from Simulink to the Sensor World.
      | 
      | - Port Name [-]: specifies the name of the output terminal of the Simulink block.
      | - Index [-]: specifies the start position in the output vector sent to the Sensor World
      | - Port dimensions [-]: specifies the width (number of scalars) of the output port
      | - Upload period [s]: specifies the upload period (in seconds) of the port.
      mask Display: port_label('input', 1, PortName)
  RPY : Subsystem  mask(ToSensorWorld){PortName=RPY_Sphere_1, PortIndex=252, PortWidth=3, TimeStep=1/100}
      mask prompts: PortName "Port Name [-]"; PortIndex "Index [-]"; PortWidth "Port Dimensions [-]"; TimeStep "Upload Period [s]"
      mask help: Sends signal(s) from Simulink to the Sensor World
      mask Help:
      | Sends signal(s) from Simulink to the Sensor World.
      | 
      | - Port Name [-]: specifies the name of the output terminal of the Simulink block.
      | - Index [-]: specifies the start position in the output vector sent to the Sensor World
      | - Port dimensions [-]: specifies the width (number of scalars) of the output port
      | - Upload period [s]: specifies the upload period (in seconds) of the port.
      mask Display: port_label('input', 1, PortName)
  Velocity : Subsystem  mask(ToSensorWorld){PortName=Velocity_Sphere_1, PortIndex=246, PortWidth=3, TimeStep=1/100}
      mask prompts: PortName "Port Name [-]"; PortIndex "Index [-]"; PortWidth "Port Dimensions [-]"; TimeStep "Upload Period [s]"
      mask help: Sends signal(s) from Simulink to the Sensor World
      mask Help:
      | Sends signal(s) from Simulink to the Sensor World.
      | 
      | - Port Name [-]: specifies the name of the output terminal of the Simulink block.
      | - Index [-]: specifies the start position in the output vector sent to the Sensor World
      | - Port dimensions [-]: specifies the width (number of scalars) of the output port
      | - Upload period [s]: specifies the upload period (in seconds) of the port.
      mask Display: port_label('input', 1, PortName)
  iniBODYAngles wrtVEH [rad] : Constant  Value=[Roll0 Pitch0 0]  SampleTime=TimeStep
  iniVEHAngles wrtGLOB [rad] : Constant  Value=[0 0 Yaw0]  SampleTime=TimeStep
  iniVEHposition wrtGLOB [m] : Constant  Value=[x0 y0 z0]  SampleTime=TimeStep
  state2FullState : PreScanSimulinkLibrary/state2FullState  SystemSampleTime=-1
  velRPY : Subsystem  mask(ToSensorWorld){PortName=velRPY_Sphere_1, PortIndex=255, PortWidth=3, TimeStep=1/100}
      mask prompts: PortName "Port Name [-]"; PortIndex "Index [-]"; PortWidth "Port Dimensions [-]"; TimeStep "Upload Period [s]"
      mask help: Sends signal(s) from Simulink to the Sensor World
      mask Help:
      | Sends signal(s) from Simulink to the Sensor World.
      | 
      | - Port Name [-]: specifies the name of the output terminal of the Simulink block.
      | - Index [-]: specifies the start position in the output vector sent to the Sensor World
      | - Port dimensions [-]: specifies the width (number of scalars) of the output port
      | - Upload period [s]: specifies the upload period (in seconds) of the port.
      mask Display: port_label('input', 1, PortName)
  wires:
  Demux/5 -> velRPY/1(Y)
  Demux/4 -> RPY/1(Y)
  Demux/3 -> Acceleration/1(Y)
  Demux/2 -> Velocity/1(Y)
  Demux/1 -> Position/1(Y)
  State/1 -> state2FullState/1
  state2FullState/1 -> Demux/1
  iniVEHposition wrtGLOB [m]/1 -> state2FullState/2
  iniBODYAngles wrtVEH [rad]/1 -> state2FullState/3
  iniVEHAngles wrtGLOB [rad]/1 -> state2FullState/4

== system NHTSA_LDW_Curved_dashed_right_cs/SetActuators ==
  Bus Creator : BusCreator  Inputs=1
  Data Store Read : DataStoreRead  DataStoreName=SimCoreActuators  SampleTime=TimeStep
  SendActuators : M-S-Function  FunctionName=SendActuatorsBlock  Parameters=TimeStep NrOfActuators
  dummy : Outport
  tag scope: SimCoreInfo=global
  wires:
  Bus Creator/1 -> [SimCoreInfo]  "SimCore"
  SendActuators/2 -> Bus Creator/1  "ComputationTime[s]"
  SendActuators/1 -> dummy/1
  Data Store Read/1 -> SendActuators/1

== system NHTSA_LDW_Curved_dashed_right_cs/SimCoreInfo ==
  Bus Selector : BusSelector  OutputSignals=ComputationTime[s]
  Time : Scope
      settings: TimeRange=10  YMin=0  YMax=0.5  SaveName=ComputationTime
  wires:
  Bus Selector/1 -> Time/1  "<ComputationTime[s]>"
  [SimCoreInfo] -> Bus Selector/1

== system NHTSA_LDW_Curved_dashed_right_cs/Sphere_1 ==
  SELF_Sphere_1 : Inport  Tag=SELFInport
  Dynamics_Empty : Subsystem  Tag=Dynamics_Empty
      mask Display: port_label('output', 1, 'State');text(0,0,' Empty\n')
  Gain : Gain  Gain=[1 1 1 1 1 1 0 0 1]
  SELF_Demux : Subsystem  Tag=DemuxSELF
      settings: DeleteFcn=PreScanBlockDeleteFcn;
      mask Type: PreScan Demux Block:
      mask Display:
      | port_label('output',1,'x [m]')
      | port_label('output',2,'y [m]')
      | port_label('output',3,'z [m]','texmode','on')
      | port_label('output',4,'Rotx [deg]','texmode','on')
      | port_label('output',5,'Roty [deg]','texmode','on')
      | port_label('output',6,'Rotz [deg]','texmode','on')
      | port_label('output',7,'GPS lat [deg]','texmode','on')
      | port_label('output',8,'GPS long [deg]','texmode','on')
      | port_label('output',9,'GPS alt [m]','texmode','on')
      | port_label('output',10,'Velocity [m/s]')
      | port_label('output',11,'Heading [deg]')
      | port_label('output',12,'Yaw rate [deg/s]')
  Terminator_{1..13} (13 alike) : Terminator
  STATE_Sphere_1 : Outport  Tag=StateOutport
  wires:
  [State] -> Gain/1
  SELF_Sphere_1/1 -> SELF_Demux/1(SELF)
  Gain/1 -> STATE_Sphere_1/1
  Dynamics_Empty/1(State) -> Terminator_1/1
  SELF_Demux/1(x [m]) -> Terminator_2/1
  SELF_Demux/2(y [m]) -> Terminator_3/1
  SELF_Demux/3(z [m]) -> Terminator_4/1
  SELF_Demux/4(rotx [deg]) -> Terminator_5/1
  SELF_Demux/5(roty [deg]) -> Terminator_6/1
  SELF_Demux/6(rotz [deg]) -> Terminator_7/1
  SELF_Demux/7(GPS lat [deg]) -> Terminator_8/1
  SELF_Demux/8(GPS long [deg]) -> Terminator_9/1
  SELF_Demux/9(GPS alt [m]) -> Terminator_10/1
  SELF_Demux/10(velocity [m/s]) -> Terminator_11/1
  SELF_Demux/11(heading [deg]) -> Terminator_12/1
  SELF_Demux/12(yaw rate [deg/s]) -> Terminator_13/1
